simulink model "CPM_V3"  (R2023a)
settings: Solver=VariableStepAuto  StartTime=0.0  StopTime=6  RelTol=1e-3
values from neighbouring files (symbols this model uses):
  A = sqrt(2*E/sampleTime)    [dataCPM.m]
  sampleTime = 1    [dataCPM.m]
undefined symbols (not defined in the file or in its folder): A_rt
libraries: simulink_extras x24, dspsigops x8, commdigbbndcpm2 x2
settings Model: Creator=mluser  LastModifiedBy=x
settings DebuggingCC: ParameterOverflowMsg=none  ParameterUnderflowMsg=error

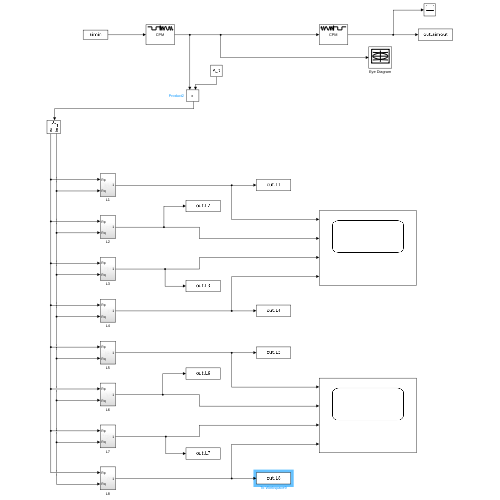
[thumbnail: Simulink's stored preview of the top-level diagram]
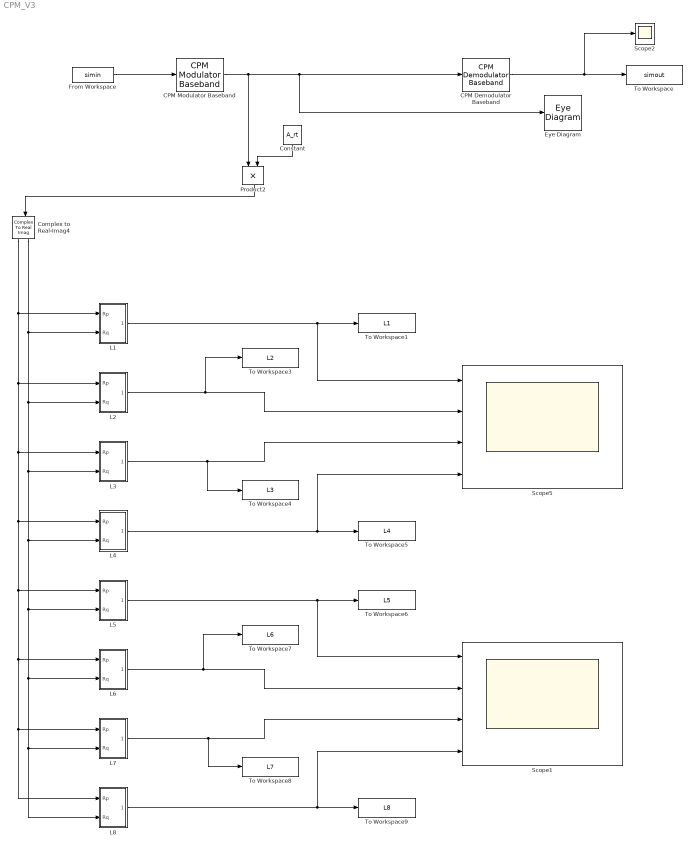
== system CPM_V3 ==
  CPM Demodulator Baseband : commdigbbndcpm2/CPM Demodulator Baseband  Mnum=2  outputType=Integer  mappingType=Binary  modIdx=0.5  pulseShape=Rectangular  BT=0.3  mainLobePulseLength=1  rollOff=0.2  pulseLength=1  preHistory=1  phaseOffset=0  samplesPerSymbol=sample_n  RateOptions=Allow multirate processing  traceBack=1  outDType=double
  CPM Modulator Baseband : commdigbbndcpm2/CPM Modulator Baseband  Mnum=2  inputType=Integer  mappingType=Binary  modIdx=0.5  pulseShape=Rectangular  BT=0.3  mainLobePulseLength=1  rollOff=0.2  pulseLength=1  preHistory=1  phaseOffset=0  samplesPerSymbol=sample_n  RateOptions=Allow multirate processing  outDataType=double
  Complex to Real-Imag4 : ComplexToRealImag
  Constant : Constant  Value=A_rt
  Eye Diagram : EyeDiagram
  From Workspace : FromWorkspace  VariableName=simin  OutDataTypeStr=double  SampleTime=sampleTime  Interpolate=off  OutputAfterFinalValue=Holding final value
  L1 : Subsystem
  L2 : Subsystem
  L3 : Subsystem
  L4 : Subsystem
  L5 : Subsystem
  L6 : Subsystem
  L7 : Subsystem
  L8 : Subsystem
  Product2 : Product
  Scope1 : Scope  NumInputPorts=4
  Scope2 : Scope
  Scope5 : Scope  NumInputPorts=4
  To Workspace : ToWorkspace  VariableName=simout  SampleTime=-1
      settings: Save2DSignal=2-D array (concatenate along first dimension)
  To Workspace1 : ToWorkspace  VariableName=L1  SampleTime=sampleTime
      settings: Save2DSignal=2-D array (concatenate along first dimension)
  To Workspace3 : ToWorkspace  VariableName=L2  SampleTime=sampleTime
      settings: Save2DSignal=2-D array (concatenate along first dimension)
  To Workspace4 : ToWorkspace  VariableName=L3  SampleTime=sampleTime
      settings: Save2DSignal=2-D array (concatenate along first dimension)
  To Workspace5 : ToWorkspace  VariableName=L4  SampleTime=sampleTime
      settings: Save2DSignal=2-D array (concatenate along first dimension)
  To Workspace6 : ToWorkspace  VariableName=L5  SampleTime=sampleTime
      settings: Save2DSignal=2-D array (concatenate along first dimension)
  To Workspace7 : ToWorkspace  VariableName=L6  SampleTime=sampleTime
      settings: Save2DSignal=2-D array (concatenate along first dimension)
  To Workspace8 : ToWorkspace  VariableName=L7  SampleTime=sampleTime
      settings: Save2DSignal=2-D array (concatenate along first dimension)
  To Workspace9 : ToWorkspace  VariableName=L8  SampleTime=sampleTime
      settings: Save2DSignal=2-D array (concatenate along first dimension)
  wires:
  From Workspace/1 -> CPM Modulator Baseband/1
  CPM Demodulator Baseband/1 -> To Workspace/1, Scope2/1
  CPM Modulator Baseband/1 -> Eye Diagram/1, CPM Demodulator Baseband/1, Product2/1
  Constant/1 -> Product2/2
  Product2/1 -> Complex to Real-Imag4/1
  L1/1(Out1) -> To Workspace1/1, Scope5/1
  L2/1(Out1) -> To Workspace3/1, Scope5/2
  Complex to Real-Imag4/1 -> L8/1(Rp), L7/1(Rp), L6/1(Rp), L5/1(Rp), L4/1(Rp), L3/1(Rp), L2/1(Rp), L1/1(Rp)
  Complex to Real-Imag4/2 -> L8/2(Rq), L7/2(Rq), L6/2(Rq), L5/2(Rq), L4/2(Rq), L3/2(Rq), L2/2(Rq), L1/2(Rq)
  L3/1(Out1) -> Scope5/3, To Workspace4/1
  L4/1(Out1) -> To Workspace5/1, Scope5/4
  L5/1(Out1) -> Scope1/1, To Workspace6/1
  L6/1(Out1) -> To Workspace7/1, Scope1/2
  L7/1(Out1) -> To Workspace8/1, Scope1/3
  L8/1(Out1) -> To Workspace9/1, Scope1/4

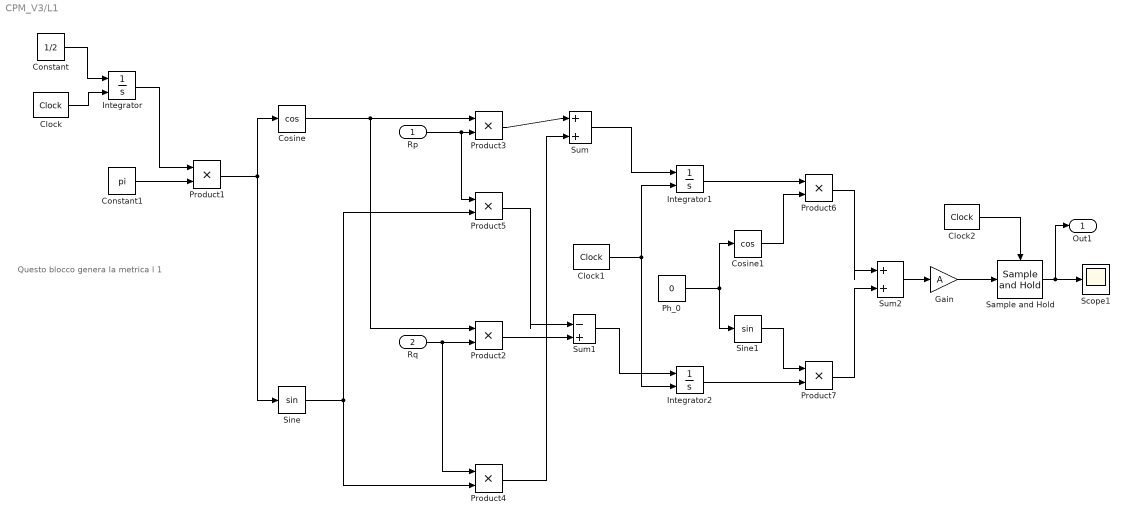
== system CPM_V3/L1 ==
  note: Questo blocco genera la metrica l 1
  Rp : Inport
  Rq : Inport  Port=2
  Clock : simulink_extras/Flip Flops/Clock  period=1
  Clock1 : simulink_extras/Flip Flops/Clock  period=sampleTime+0.00000001
  Clock2 : simulink_extras/Flip Flops/Clock  period=1
  Constant : Constant  Value=1/2
  Constant1 : Constant  Value=pi
  Cosine : Trigonometry  Operator=cos  NumberOfIterations=32  NumberOfDataPoints=32
  Cosine1 : Trigonometry  Operator=cos  NumberOfIterations=32  NumberOfDataPoints=32
  Gain : Gain  Gain=A
  Integrator : Integrator  ExternalReset=rising
  Integrator1 : Integrator  ExternalReset=rising
  Integrator2 : Integrator  ExternalReset=rising
  Ph_0 : Constant  Value=0
  Product{1..7} (7 alike) : Product
  Sample and Hold : dspsigops/Sample and Hold  trig=Rising edge  initCond=0  latchinput=off
  Scope1 : Scope
  Sine : Trigonometry  NumberOfIterations=32  NumberOfDataPoints=32
  Sine1 : Trigonometry  NumberOfIterations=32  NumberOfDataPoints=32
  Sum : Sum  Inputs=|++
  Sum1 : Sum  Inputs=|-+
  Sum2 : Sum  Inputs=|++
  Out1 : Outport
  wires:
  Rq/1 -> Product4/1, Product2/2
  Rp/1 -> Product5/1, Product3/2
  Integrator/1 -> Product1/1
  Cosine/1 -> Product3/1, Product2/1
  Sine/1 -> Product5/2, Product4/2
  Constant1/1 -> Product1/2
  Constant/1 -> Integrator/1
  Clock/1 -> Integrator/2
  Sum/1 -> Integrator1/1
  Product1/1 -> Sine/1, Cosine/1
  Product3/1 -> Sum/1
  Product4/1 -> Sum/2
  Clock1/1 -> Integrator2/2, Integrator1/2
  Sum1/1 -> Integrator2/1
  Ph_0/1 -> Cosine1/1, Sine1/1
  Integrator1/1 -> Product6/1
  Integrator2/1 -> Product7/2
  Sine1/1 -> Product7/1
  Cosine1/1 -> Product6/2
  Sum2/1 -> Gain/1
  Product6/1 -> Sum2/1
  Product7/1 -> Sum2/2
  Product5/1 -> Sum1/1
  Product2/1 -> Sum1/2
  Sample and Hold/1 -> Out1/1, Scope1/1
  Gain/1 -> Sample and Hold/1
  Clock2/1 -> Sample and Hold/Trigger

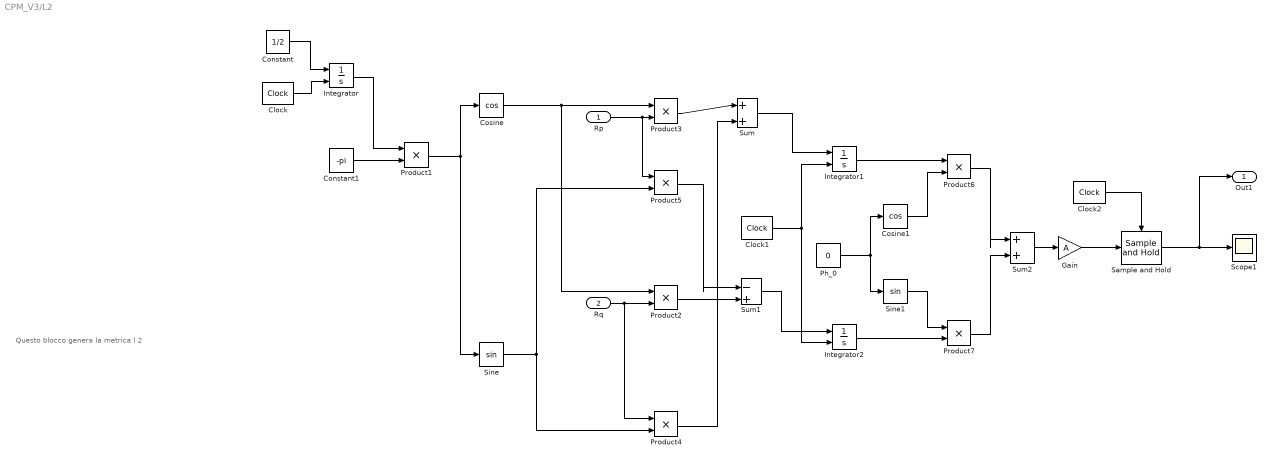
== system CPM_V3/L2 ==
  note: Questo blocco genera la metrica l 2
  Rp : Inport
  Rq : Inport  Port=2
  Clock : simulink_extras/Flip Flops/Clock  period=1
  Clock1 : simulink_extras/Flip Flops/Clock  period=sampleTime+0.00000001
  Clock2 : simulink_extras/Flip Flops/Clock  period=1
  Constant : Constant  Value=1/2
  Constant1 : Constant  Value=-pi
  Cosine : Trigonometry  Operator=cos  NumberOfIterations=32  NumberOfDataPoints=32
  Cosine1 : Trigonometry  Operator=cos  NumberOfIterations=32  NumberOfDataPoints=32
  Gain : Gain  Gain=A
  Integrator : Integrator  ExternalReset=rising
  Integrator1 : Integrator  ExternalReset=rising
  Integrator2 : Integrator  ExternalReset=rising
  Ph_0 : Constant  Value=0
  Product{1..7} (7 alike) : Product
  Sample and Hold : dspsigops/Sample and Hold  trig=Rising edge  initCond=0  latchinput=off
  Scope1 : Scope
  Sine : Trigonometry  NumberOfIterations=32  NumberOfDataPoints=32
  Sine1 : Trigonometry  NumberOfIterations=32  NumberOfDataPoints=32
  Sum : Sum  Inputs=|++
  Sum1 : Sum  Inputs=|-+
  Sum2 : Sum  Inputs=|++
  Out1 : Outport
  wires:
  Rq/1 -> Product4/1, Product2/2
  Rp/1 -> Product5/1, Product3/2
  Integrator/1 -> Product1/1
  Cosine/1 -> Product3/1, Product2/1
  Sine/1 -> Product5/2, Product4/2
  Constant1/1 -> Product1/2
  Constant/1 -> Integrator/1
  Clock/1 -> Integrator/2
  Sum/1 -> Integrator1/1
  Product1/1 -> Sine/1, Cosine/1
  Product3/1 -> Sum/1
  Product4/1 -> Sum/2
  Clock1/1 -> Integrator2/2, Integrator1/2
  Sum1/1 -> Integrator2/1
  Ph_0/1 -> Cosine1/1, Sine1/1
  Integrator1/1 -> Product6/1
  Integrator2/1 -> Product7/2
  Sine1/1 -> Product7/1
  Cosine1/1 -> Product6/2
  Sum2/1 -> Gain/1
  Product6/1 -> Sum2/1
  Product7/1 -> Sum2/2
  Product5/1 -> Sum1/1
  Product2/1 -> Sum1/2
  Clock2/1 -> Sample and Hold/Trigger
  Gain/1 -> Sample and Hold/1
  Sample and Hold/1 -> Out1/1, Scope1/1

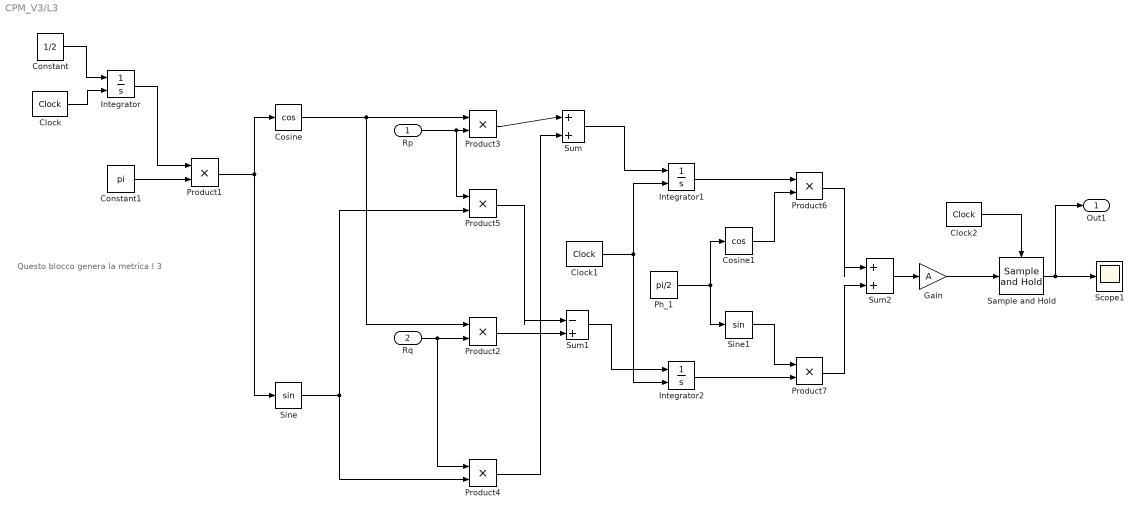
== system CPM_V3/L3 ==
  note: Questo blocco genera la metrica l 3
  Rp : Inport
  Rq : Inport  Port=2
  Clock : simulink_extras/Flip Flops/Clock  period=1
  Clock1 : simulink_extras/Flip Flops/Clock  period=sampleTime+0.00000001
  Clock2 : simulink_extras/Flip Flops/Clock  period=1
  Constant : Constant  Value=1/2
  Constant1 : Constant  Value=pi
  Cosine : Trigonometry  Operator=cos  NumberOfIterations=32  NumberOfDataPoints=32
  Cosine1 : Trigonometry  Operator=cos  NumberOfIterations=32  NumberOfDataPoints=32
  Gain : Gain  Gain=A
  Integrator : Integrator  ExternalReset=rising
  Integrator1 : Integrator  ExternalReset=rising
  Integrator2 : Integrator  ExternalReset=rising
  Ph_1 : Constant  Value=pi/2
  Product{1..7} (7 alike) : Product
  Sample and Hold : dspsigops/Sample and Hold  trig=Rising edge  initCond=0  latchinput=off
  Scope1 : Scope
  Sine : Trigonometry  NumberOfIterations=32  NumberOfDataPoints=32
  Sine1 : Trigonometry  NumberOfIterations=32  NumberOfDataPoints=32
  Sum : Sum  Inputs=|++
  Sum1 : Sum  Inputs=|-+
  Sum2 : Sum  Inputs=|++
  Out1 : Outport
  wires:
  Rq/1 -> Product4/1, Product2/2
  Rp/1 -> Product5/1, Product3/2
  Integrator/1 -> Product1/1
  Cosine/1 -> Product3/1, Product2/1
  Sine/1 -> Product5/2, Product4/2
  Constant1/1 -> Product1/2
  Constant/1 -> Integrator/1
  Clock/1 -> Integrator/2
  Sum/1 -> Integrator1/1
  Product1/1 -> Sine/1, Cosine/1
  Product3/1 -> Sum/1
  Product4/1 -> Sum/2
  Clock1/1 -> Integrator2/2, Integrator1/2
  Sum1/1 -> Integrator2/1
  Ph_1/1 -> Cosine1/1, Sine1/1
  Integrator1/1 -> Product6/1
  Integrator2/1 -> Product7/2
  Sine1/1 -> Product7/1
  Cosine1/1 -> Product6/2
  Sum2/1 -> Gain/1
  Product6/1 -> Sum2/1
  Product7/1 -> Sum2/2
  Product5/1 -> Sum1/1
  Product2/1 -> Sum1/2
  Clock2/1 -> Sample and Hold/Trigger
  Gain/1 -> Sample and Hold/1
  Sample and Hold/1 -> Out1/1, Scope1/1

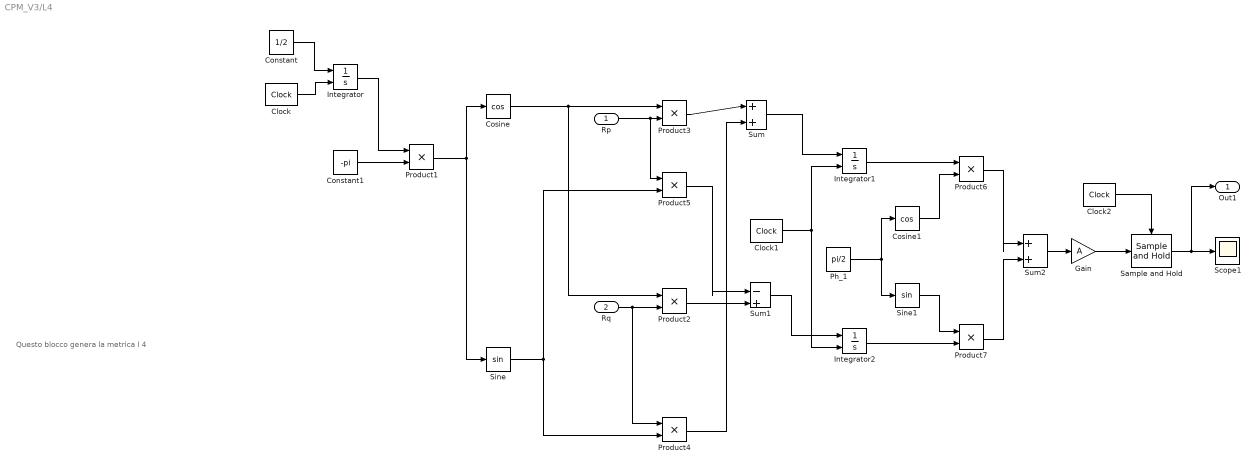
== system CPM_V3/L4 ==
  note: Questo blocco genera la metrica l 4
  Rp : Inport
  Rq : Inport  Port=2
  Clock : simulink_extras/Flip Flops/Clock  period=1
  Clock1 : simulink_extras/Flip Flops/Clock  period=sampleTime+0.00000001
  Clock2 : simulink_extras/Flip Flops/Clock  period=1
  Constant : Constant  Value=1/2
  Constant1 : Constant  Value=-pi
  Cosine : Trigonometry  Operator=cos  NumberOfIterations=32  NumberOfDataPoints=32
  Cosine1 : Trigonometry  Operator=cos  NumberOfIterations=32  NumberOfDataPoints=32
  Gain : Gain  Gain=A
  Integrator : Integrator  ExternalReset=rising
  Integrator1 : Integrator  ExternalReset=rising
  Integrator2 : Integrator  ExternalReset=rising
  Ph_1 : Constant  Value=pi/2
  Product{1..7} (7 alike) : Product
  Sample and Hold : dspsigops/Sample and Hold  trig=Rising edge  initCond=0  latchinput=off
  Scope1 : Scope
  Sine : Trigonometry  NumberOfIterations=32  NumberOfDataPoints=32
  Sine1 : Trigonometry  NumberOfIterations=32  NumberOfDataPoints=32
  Sum : Sum  Inputs=|++
  Sum1 : Sum  Inputs=|-+
  Sum2 : Sum  Inputs=|++
  Out1 : Outport
  wires:
  Rq/1 -> Product4/1, Product2/2
  Rp/1 -> Product5/1, Product3/2
  Integrator/1 -> Product1/1
  Cosine/1 -> Product3/1, Product2/1
  Sine/1 -> Product5/2, Product4/2
  Constant1/1 -> Product1/2
  Constant/1 -> Integrator/1
  Clock/1 -> Integrator/2
  Sum/1 -> Integrator1/1
  Product1/1 -> Sine/1, Cosine/1
  Product3/1 -> Sum/1
  Product4/1 -> Sum/2
  Clock1/1 -> Integrator2/2, Integrator1/2
  Sum1/1 -> Integrator2/1
  Ph_1/1 -> Cosine1/1, Sine1/1
  Integrator1/1 -> Product6/1
  Integrator2/1 -> Product7/2
  Sine1/1 -> Product7/1
  Cosine1/1 -> Product6/2
  Sum2/1 -> Gain/1
  Product6/1 -> Sum2/1
  Product7/1 -> Sum2/2
  Product5/1 -> Sum1/1
  Product2/1 -> Sum1/2
  Clock2/1 -> Sample and Hold/Trigger
  Gain/1 -> Sample and Hold/1
  Sample and Hold/1 -> Out1/1, Scope1/1

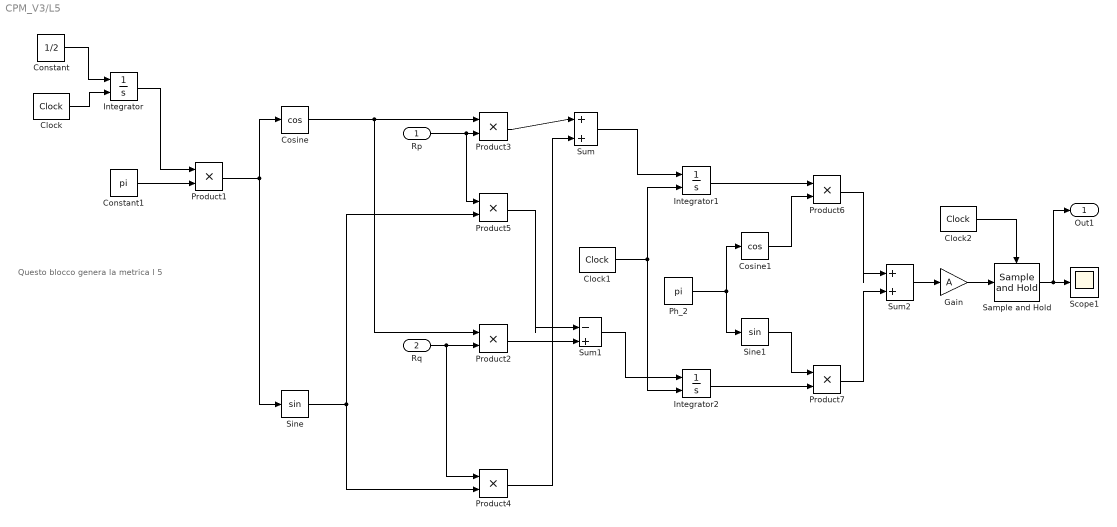
== system CPM_V3/L5 ==
  note: Questo blocco genera la metrica l 5
  Rp : Inport
  Rq : Inport  Port=2
  Clock : simulink_extras/Flip Flops/Clock  period=1
  Clock1 : simulink_extras/Flip Flops/Clock  period=sampleTime+0.00000001
  Clock2 : simulink_extras/Flip Flops/Clock  period=1
  Constant : Constant  Value=1/2
  Constant1 : Constant  Value=pi
  Cosine : Trigonometry  Operator=cos  NumberOfIterations=32  NumberOfDataPoints=32
  Cosine1 : Trigonometry  Operator=cos  NumberOfIterations=32  NumberOfDataPoints=32
  Gain : Gain  Gain=A
  Integrator : Integrator  ExternalReset=rising
  Integrator1 : Integrator  ExternalReset=rising
  Integrator2 : Integrator  ExternalReset=rising
  Ph_2 : Constant  Value=pi
  Product{1..7} (7 alike) : Product
  Sample and Hold : dspsigops/Sample and Hold  trig=Rising edge  initCond=0  latchinput=off
  Scope1 : Scope
  Sine : Trigonometry  NumberOfIterations=32  NumberOfDataPoints=32
  Sine1 : Trigonometry  NumberOfIterations=32  NumberOfDataPoints=32
  Sum : Sum  Inputs=|++
  Sum1 : Sum  Inputs=|-+
  Sum2 : Sum  Inputs=|++
  Out1 : Outport
  wires:
  Rq/1 -> Product4/1, Product2/2
  Rp/1 -> Product5/1, Product3/2
  Integrator/1 -> Product1/1
  Cosine/1 -> Product3/1, Product2/1
  Sine/1 -> Product5/2, Product4/2
  Constant1/1 -> Product1/2
  Constant/1 -> Integrator/1
  Clock/1 -> Integrator/2
  Sum/1 -> Integrator1/1
  Product1/1 -> Sine/1, Cosine/1
  Product3/1 -> Sum/1
  Product4/1 -> Sum/2
  Clock1/1 -> Integrator2/2, Integrator1/2
  Sum1/1 -> Integrator2/1
  Ph_2/1 -> Cosine1/1, Sine1/1
  Integrator1/1 -> Product6/1
  Integrator2/1 -> Product7/2
  Sine1/1 -> Product7/1
  Cosine1/1 -> Product6/2
  Sum2/1 -> Gain/1
  Product6/1 -> Sum2/1
  Product7/1 -> Sum2/2
  Product5/1 -> Sum1/1
  Product2/1 -> Sum1/2
  Clock2/1 -> Sample and Hold/Trigger
  Gain/1 -> Sample and Hold/1
  Sample and Hold/1 -> Out1/1, Scope1/1

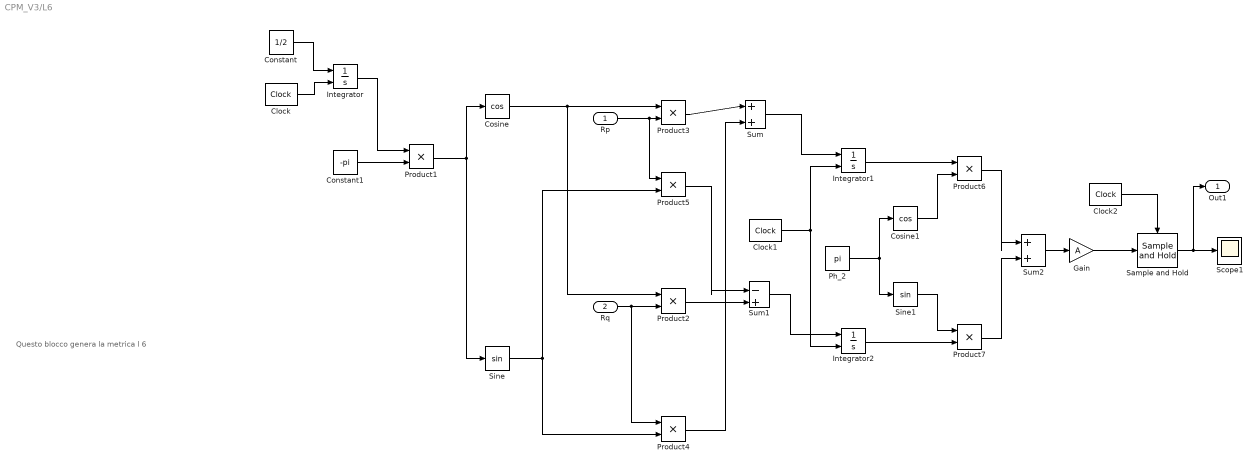
== system CPM_V3/L6 ==
  note: Questo blocco genera la metrica l 6
  Rp : Inport
  Rq : Inport  Port=2
  Clock : simulink_extras/Flip Flops/Clock  period=1
  Clock1 : simulink_extras/Flip Flops/Clock  period=sampleTime+0.00000001
  Clock2 : simulink_extras/Flip Flops/Clock  period=1
  Constant : Constant  Value=1/2
  Constant1 : Constant  Value=-pi
  Cosine : Trigonometry  Operator=cos  NumberOfIterations=32  NumberOfDataPoints=32
  Cosine1 : Trigonometry  Operator=cos  NumberOfIterations=32  NumberOfDataPoints=32
  Gain : Gain  Gain=A
  Integrator : Integrator  ExternalReset=rising
  Integrator1 : Integrator  ExternalReset=rising
  Integrator2 : Integrator  ExternalReset=rising
  Ph_2 : Constant  Value=pi
  Product{1..7} (7 alike) : Product
  Sample and Hold : dspsigops/Sample and Hold  trig=Rising edge  initCond=0  latchinput=off
  Scope1 : Scope
  Sine : Trigonometry  NumberOfIterations=32  NumberOfDataPoints=32
  Sine1 : Trigonometry  NumberOfIterations=32  NumberOfDataPoints=32
  Sum : Sum  Inputs=|++
  Sum1 : Sum  Inputs=|-+
  Sum2 : Sum  Inputs=|++
  Out1 : Outport
  wires:
  Rq/1 -> Product4/1, Product2/2
  Rp/1 -> Product5/1, Product3/2
  Integrator/1 -> Product1/1
  Cosine/1 -> Product3/1, Product2/1
  Sine/1 -> Product5/2, Product4/2
  Constant1/1 -> Product1/2
  Constant/1 -> Integrator/1
  Clock/1 -> Integrator/2
  Sum/1 -> Integrator1/1
  Product1/1 -> Sine/1, Cosine/1
  Product3/1 -> Sum/1
  Product4/1 -> Sum/2
  Clock1/1 -> Integrator2/2, Integrator1/2
  Sum1/1 -> Integrator2/1
  Ph_2/1 -> Cosine1/1, Sine1/1
  Integrator1/1 -> Product6/1
  Integrator2/1 -> Product7/2
  Sine1/1 -> Product7/1
  Cosine1/1 -> Product6/2
  Sum2/1 -> Gain/1
  Product6/1 -> Sum2/1
  Product7/1 -> Sum2/2
  Product5/1 -> Sum1/1
  Product2/1 -> Sum1/2
  Clock2/1 -> Sample and Hold/Trigger
  Gain/1 -> Sample and Hold/1
  Sample and Hold/1 -> Out1/1, Scope1/1

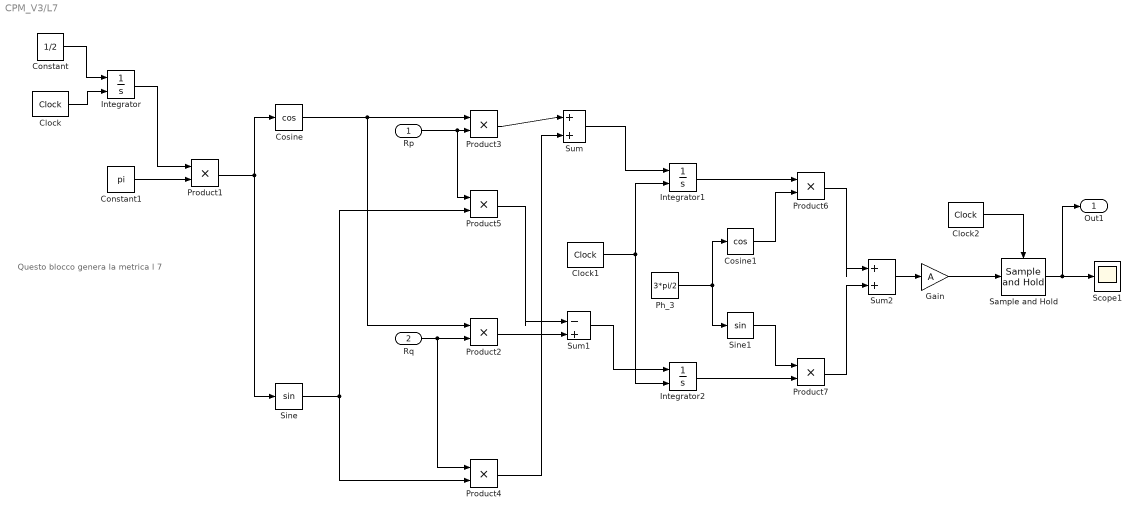
== system CPM_V3/L7 ==
  note: Questo blocco genera la metrica l 7
  Rp : Inport
  Rq : Inport  Port=2
  Clock : simulink_extras/Flip Flops/Clock  period=1
  Clock1 : simulink_extras/Flip Flops/Clock  period=sampleTime+0.00000001
  Clock2 : simulink_extras/Flip Flops/Clock  period=1
  Constant : Constant  Value=1/2
  Constant1 : Constant  Value=pi
  Cosine : Trigonometry  Operator=cos  NumberOfIterations=32  NumberOfDataPoints=32
  Cosine1 : Trigonometry  Operator=cos  NumberOfIterations=32  NumberOfDataPoints=32
  Gain : Gain  Gain=A
  Integrator : Integrator  ExternalReset=rising
  Integrator1 : Integrator  ExternalReset=rising
  Integrator2 : Integrator  ExternalReset=rising
  Ph_3 : Constant  Value=3*pi/2
  Product{1..7} (7 alike) : Product
  Sample and Hold : dspsigops/Sample and Hold  trig=Rising edge  initCond=0  latchinput=off
  Scope1 : Scope
  Sine : Trigonometry  NumberOfIterations=32  NumberOfDataPoints=32
  Sine1 : Trigonometry  NumberOfIterations=32  NumberOfDataPoints=32
  Sum : Sum  Inputs=|++
  Sum1 : Sum  Inputs=|-+
  Sum2 : Sum  Inputs=|++
  Out1 : Outport
  wires:
  Rq/1 -> Product4/1, Product2/2
  Rp/1 -> Product5/1, Product3/2
  Integrator/1 -> Product1/1
  Cosine/1 -> Product3/1, Product2/1
  Sine/1 -> Product5/2, Product4/2
  Constant1/1 -> Product1/2
  Constant/1 -> Integrator/1
  Clock/1 -> Integrator/2
  Sum/1 -> Integrator1/1
  Product1/1 -> Sine/1, Cosine/1
  Product3/1 -> Sum/1
  Product4/1 -> Sum/2
  Clock1/1 -> Integrator2/2, Integrator1/2
  Sum1/1 -> Integrator2/1
  Ph_3/1 -> Cosine1/1, Sine1/1
  Integrator1/1 -> Product6/1
  Integrator2/1 -> Product7/2
  Sine1/1 -> Product7/1
  Cosine1/1 -> Product6/2
  Sum2/1 -> Gain/1
  Product6/1 -> Sum2/1
  Product7/1 -> Sum2/2
  Product5/1 -> Sum1/1
  Product2/1 -> Sum1/2
  Clock2/1 -> Sample and Hold/Trigger
  Gain/1 -> Sample and Hold/1
  Sample and Hold/1 -> Out1/1, Scope1/1

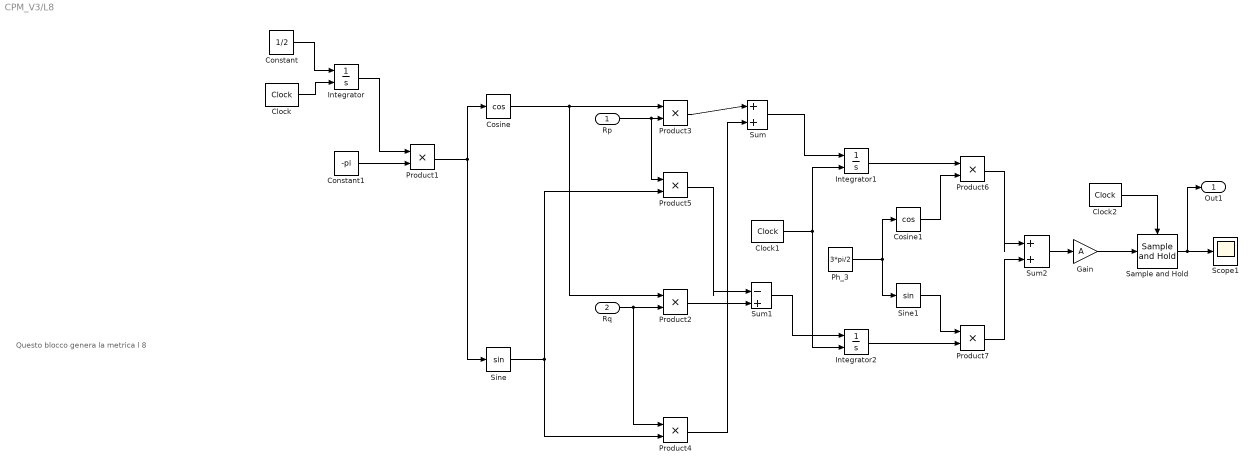
== system CPM_V3/L8 ==
  note: Questo blocco genera la metrica l 8
  Rp : Inport
  Rq : Inport  Port=2
  Clock : simulink_extras/Flip Flops/Clock  period=1
  Clock1 : simulink_extras/Flip Flops/Clock  period=sampleTime+0.00000001
  Clock2 : simulink_extras/Flip Flops/Clock  period=1
  Constant : Constant  Value=1/2
  Constant1 : Constant  Value=-pi
  Cosine : Trigonometry  Operator=cos  NumberOfIterations=32  NumberOfDataPoints=32
  Cosine1 : Trigonometry  Operator=cos  NumberOfIterations=32  NumberOfDataPoints=32
  Gain : Gain  Gain=A
  Integrator : Integrator  ExternalReset=rising
  Integrator1 : Integrator  ExternalReset=rising
  Integrator2 : Integrator  ExternalReset=rising
  Ph_3 : Constant  Value=3*pi/2
  Product{1..7} (7 alike) : Product
  Sample and Hold : dspsigops/Sample and Hold  trig=Rising edge  initCond=0  latchinput=off
  Scope1 : Scope
  Sine : Trigonometry  NumberOfIterations=32  NumberOfDataPoints=32
  Sine1 : Trigonometry  NumberOfIterations=32  NumberOfDataPoints=32
  Sum : Sum  Inputs=|++
  Sum1 : Sum  Inputs=|-+
  Sum2 : Sum  Inputs=|++
  Out1 : Outport
  wires:
  Rq/1 -> Product4/1, Product2/2
  Rp/1 -> Product5/1, Product3/2
  Integrator/1 -> Product1/1
  Cosine/1 -> Product3/1, Product2/1
  Sine/1 -> Product5/2, Product4/2
  Constant1/1 -> Product1/2
  Constant/1 -> Integrator/1
  Clock/1 -> Integrator/2
  Sum/1 -> Integrator1/1
  Product1/1 -> Sine/1, Cosine/1
  Product3/1 -> Sum/1
  Product4/1 -> Sum/2
  Clock1/1 -> Integrator2/2, Integrator1/2
  Sum1/1 -> Integrator2/1
  Ph_3/1 -> Cosine1/1, Sine1/1
  Integrator1/1 -> Product6/1
  Integrator2/1 -> Product7/2
  Sine1/1 -> Product7/1
  Cosine1/1 -> Product6/2
  Sum2/1 -> Gain/1
  Product6/1 -> Sum2/1
  Product7/1 -> Sum2/2
  Product5/1 -> Sum1/1
  Product2/1 -> Sum1/2
  Clock2/1 -> Sample and Hold/Trigger
  Gain/1 -> Sample and Hold/1
  Sample and Hold/1 -> Out1/1, Scope1/1
